simulink model "MSD2"  (R2016a)
settings: Solver=ode45  StartTime=0.0  StopTime=10  RelTol=1e-6
model workspace (MAT data in the model file):
  C = 2
  D = 2
  m = 2
settings Model: Creator=METZLER  LastModifiedBy=chris.barlow
settings DataIOCC: LimitDataPoints=on  SaveFormat=Array  SignalLoggingSaveFormat=ModelDataLogs
settings OptimizationCC: InitFltsAndDblsToZero=on
settings DebuggingCC: SaveWithParameterizedLinksMsg=none  UnderspecifiedInitializationDetection=Classic  MergeDetectMultiDrivingBlocksExec=none  SignalResolutionControl=TryResolveAllWithWarning  SolverPrmCheckMsg=warning  MultiTaskDSMMsg=warning  MultiTaskCondExecSysMsg=none  FcnCallInpInsideContextMsg=UseLocalSettings  AllowSymbolicDim=off
settings HardwareCC: ProdBitPerPointer=32  ProdLargestAtomicFloat=None  ProdIntDivRoundTo=Undefined  ProdEndianess=Unspecified  ProdWordSize=32  ProdHWDeviceType=32-bit Generic
settings ModelReferenceCC: PropagateSignalLabelsOutOfModel=off
settings GRTTargetCC: TargetFcnLib=ansi_tfl_tmw.mat  GeneratePreprocessorConditionals=Use local settings  CombineOutputUpdateFcns=off  GRTInterface=on
settings ConfigComp: CovModelRefEnable=Off

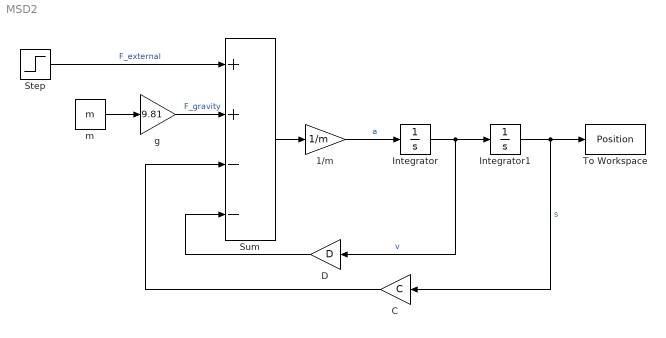
== system MSD2 ==
  1/m : Gain  Gain=1/m
  C : Gain  Gain=C
  D : Gain  Gain=D
  Integrator : Integrator
  Integrator1 : Integrator
  Step : Step  Time=0  After=10  SampleTime=0
  Sum : Sum  Inputs=++--
  To Workspace : ToWorkspace  VariableName=Position  SaveFormat=Structure With Time  SampleTime=-1
  g : Gain  Gain=9.81
  m : Constant  Value=m
  wires:
  Integrator/1 -> Integrator1/1, D/1  "v"
  Integrator1/1 -> C/1, To Workspace/1  "s"
  1/m/1 -> Integrator/1  "a"
  D/1 -> Sum/4
  g/1 -> Sum/2  "F_gravity"
  m/1 -> g/1
  Sum/1 -> 1/m/1
  C/1 -> Sum/3
  Step/1 -> Sum/1  "F_external"
